simulink model "feng_unpack"  (R2012b)
settings: Solver=FixedStepDiscrete  SolverMode=SingleTasking  StartTime=0.0  StopTime=1500000  RelTol=1e-3
undefined symbols (not defined in the file or in its folder): Down, Up
libraries: xbsIndex_r4 x1511, simulink x1, xps_library x1
(part 3 of 13)

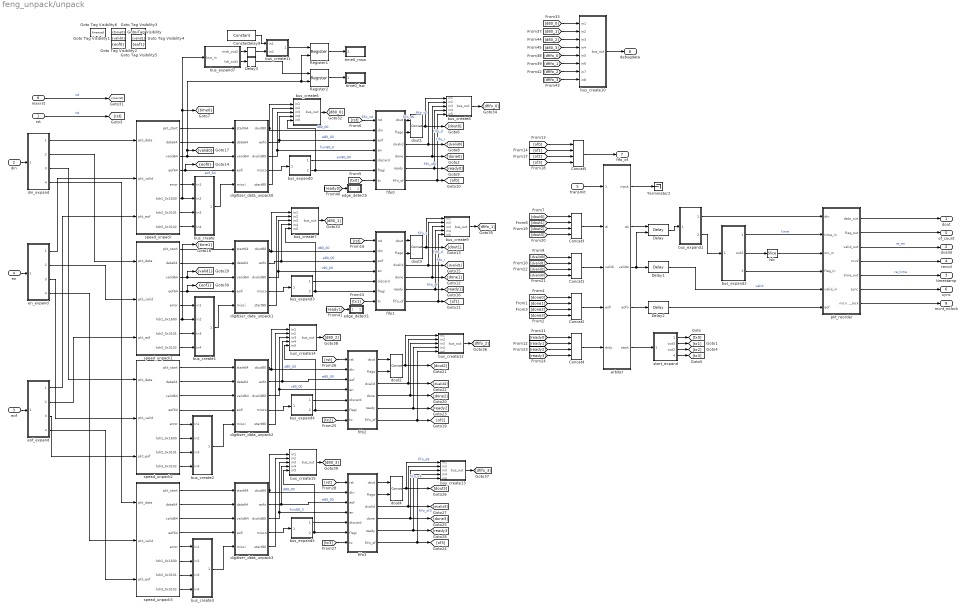
== system feng_unpack/unpack ==
  rst : Inport
  din : Inport  Port=2
  eof : Inport  Port=3
  en : Inport  Port=4
  transmit : Inport  Port=5
  maxrst : Inport  Port=6
  Concat{1..5} (5 alike) : xbsIndex_r4/Concat  num_inputs=4  dbl_ovrd=off  block_type=concat
  Constant : xbsIndex_r4/Constant  const=762.331  gui_display_data_type=Fixed-point  arith_type=Signed (2's comp)  n_bits=16  bin_pt=5  preci_type=Single  exp_width=8  frac_width=24  explicit_period=on  period=1  equ=P=C  opselect=C  inp2=PCIN>>17  opr=+  inp1=P  carry=CIN  dbl_ovrd=off  block_type=constant
  Delay : xbsIndex_r4/Delay  rst=off  infoeditControl=Selection of Reset will increase slice count due to use of real FFs and instead of SRLs  en=on  latency=1  dbl_ovrd=off  reg_retiming=on  block_type=delay
  Delay1 : xbsIndex_r4/Delay  rst=off  infoeditControl=Selection of Reset will increase slice count due to use of real FFs and instead of SRLs  en=off  latency=1  dbl_ovrd=off  reg_retiming=on  block_type=delay
  Delay2 : xbsIndex_r4/Delay  rst=off  infoeditControl=Selection of Reset will increase slice count due to use of real FFs and instead of SRLs  en=off  latency=1  dbl_ovrd=off  reg_retiming=on  block_type=delay
  Delay3 : xbsIndex_r4/Delay  rst=off  infoeditControl=Selection of Reset will increase slice count due to use of real FFs and instead of SRLs  en=off  latency=1  dbl_ovrd=off  reg_retiming=off  block_type=delay
  Delay9 : xbsIndex_r4/Delay  rst=off  infoeditControl=Selection of Reset will increase slice count due to use of real FFs and instead of SRLs  en=off  latency=1  dbl_ovrd=off  reg_retiming=off  block_type=delay
  Goto Tag Visibility : GotoTagVisibility  GotoTag=time0
  Goto Tag Visibility1 : GotoTagVisibility  GotoTag=valid0
  Goto Tag Visibility2 : GotoTagVisibility  GotoTag=eof0
  Goto Tag Visibility3 : GotoTagVisibility  GotoTag=time1
  Goto Tag Visibility4 : GotoTagVisibility  GotoTag=valid1
  Goto Tag Visibility5 : GotoTagVisibility  GotoTag=eof1
  Goto Tag Visibility6 : GotoTagVisibility  GotoTag=maxrst
  Register1 : xbsIndex_r4/Register  init=0  rst=off  en=on  dbl_ovrd=off  block_type=register
  Register2 : xbsIndex_r4/Register  init=0  rst=off  en=on  dbl_ovrd=off  block_type=register
  Terminator2 : Terminator
  arbiter : Subsystem  mask{n_inputs=4, n_bits_input=160 + n_bits_timestamp + n_bits_source + n_bits_of_count, mux_latency=1, preempt=1, n_bits_block_size=n_bits_packet_size-1, n_cycles_preempt=6}
      mask prompts: n_inputs "number of inputs"; n_bits_input "input bit widths"; mux_latency "mux latency"; preempt "preempt start of next block"; n_bits_block_size "data block size (2^?)"; n_cycles_preempt "clock cycles to preempt at"
      mask init:
      | set_param([gcb, '/eofi_mux'], ...
      |     'n_bits', 'ones(1, n_inputs)', ...
      |     'mux_latency', 'mux_latency', ...
      |     'cmplx', 'off', 'misc', 'off');
      | set_param([gcb, '/di_mux'], ...
      |     'n_bits', 'repmat(n_bits_input, 1, n_inputs)', ...
      |     'mux_latency', 'mux_latency', ...
      |     'cmplx', 'off', 'misc', 'off');
      | set_param([gcb, '/validi_mux'], ...
      |     'n_bits', 'ones(1, n_inputs)', ...
      |     'mux_latency', 'mux_latency', ...
      |     'cmplx', 'off', 'misc', 'off');
      | set_param([gcb, '/busy_edge_rep'], ...
      |     'replication', 'n_inputs', ...
      |     'misc', 'off');
  bus_create : Subsystem  AncestorBlock=casper_library_flow_control/bus_create  mask(bus_create){inputNum=4}
      mask prompts: inputNum "Number of inputs:"
      mask init:
      | bus_create_init(gcb,...
      |     'inputNum', inputNum);
  bus_create1 : Subsystem  AncestorBlock=casper_library_flow_control/bus_create  mask(bus_create){inputNum=4}
      mask prompts: inputNum "Number of inputs:"
      mask init:
      | bus_create_init(gcb,...
      |     'inputNum', inputNum);
  bus_create10 : Subsystem  AncestorBlock=casper_library_flow_control/bus_create  mask(bus_create){inputNum=8}
      mask prompts: inputNum "Number of inputs:"
      mask init:
      | bus_create_init(gcb,...
      |     'inputNum', inputNum);
  bus_create11 : Subsystem  AncestorBlock=casper_library_flow_control/bus_create  mask(bus_create){inputNum=2}
      mask prompts: inputNum "Number of inputs:"
      mask init:
      | bus_create_init(gcb,...
      |     'inputNum', inputNum);
  bus_create12 : Subsystem  AncestorBlock=casper_library_flow_control/bus_create  mask(bus_create){inputNum=5}
      mask prompts: inputNum "Number of inputs:"
      mask init:
      | bus_create_init(gcb,...
      |     'inputNum', inputNum);
  bus_create13 : Subsystem  AncestorBlock=casper_library_flow_control/bus_create  mask(bus_create){inputNum=5}
      mask prompts: inputNum "Number of inputs:"
      mask init:
      | bus_create_init(gcb,...
      |     'inputNum', inputNum);
  bus_create14 : Subsystem  AncestorBlock=casper_library_flow_control/bus_create  mask(bus_create){inputNum=5}
      mask prompts: inputNum "Number of inputs:"
      mask init:
      | bus_create_init(gcb,...
      |     'inputNum', inputNum);
  bus_create15 : Subsystem  AncestorBlock=casper_library_flow_control/bus_create  mask(bus_create){inputNum=5}
      mask prompts: inputNum "Number of inputs:"
      mask init:
      | bus_create_init(gcb,...
      |     'inputNum', inputNum);
  bus_create2 : Subsystem  AncestorBlock=casper_library_flow_control/bus_create  mask(bus_create){inputNum=4}
      mask prompts: inputNum "Number of inputs:"
      mask init:
      | bus_create_init(gcb,...
      |     'inputNum', inputNum);
  bus_create3 : Subsystem  AncestorBlock=casper_library_flow_control/bus_create  mask(bus_create){inputNum=4}
      mask prompts: inputNum "Number of inputs:"
      mask init:
      | bus_create_init(gcb,...
      |     'inputNum', inputNum);
  bus_create6 : Subsystem  AncestorBlock=casper_library_flow_control/bus_create  mask(bus_create){inputNum=5}
      mask prompts: inputNum "Number of inputs:"
      mask init:
      | bus_create_init(gcb,...
      |     'inputNum', inputNum);
  bus_create7 : Subsystem  AncestorBlock=casper_library_flow_control/bus_create  mask(bus_create){inputNum=5}
      mask prompts: inputNum "Number of inputs:"
      mask init:
      | bus_create_init(gcb,...
      |     'inputNum', inputNum);
  bus_create8 : Subsystem  AncestorBlock=casper_library_flow_control/bus_create  mask(bus_create){inputNum=5}
      mask prompts: inputNum "Number of inputs:"
      mask init:
      | bus_create_init(gcb,...
      |     'inputNum', inputNum);
  bus_create9 : Subsystem  AncestorBlock=casper_library_flow_control/bus_create  mask(bus_create){inputNum=5}
      mask prompts: inputNum "Number of inputs:"
      mask init:
      | bus_create_init(gcb,...
      |     'inputNum', inputNum);
  bus_expand0 : Subsystem  AncestorBlock=casper_library_flow_control/bus_expand  mask(bus_expand){mode=divisions of arbitrary size, outputNum=1, outputWidth=[1, sum([n_bits_timestamp, n_bits_source, n_bits_of_count])], outputBinaryPt=[0 0], outputArithmeticType=[2 0], show_format=on, outputToWorkspace=off, variablePrefix=out, outputToModelAsWell=on}
      mask prompts: outputNum "Number of outputs:"; outputWidth "Output width [msb ... lsb]:"; outputBinaryPt "Output binary point position [msb ... lsb]:"; outputArithmeticType "Output arithmetic type (ufix=0, fix=1, bool=2) [msb ... lsb]:"; show_format "Print format string?"; outputToWorkspace "Output to workspace?"; variablePrefix "Variable name prefix:"; outputToModelAsWell "Output to model as well?"
      mask help:
      | Expands a 'bus' made using a bus_create or Xilinx
      | concat block.
      | The input will be divided into the specified number
      | of outputs with the specified arithmetic types.
      | Divisions are made from most significant bit.
      mask init: same as feng_unpack/bus_expand10
      settings: AttributesFormatString=2 outputs: b,uf144.0,
      mask TypeOptions mode: divisions of equal size | divisions of arbitrary size
      mask Callback mode: bus_expand_callback();
      mask Callback outputWidth: bus_expand_callback();
      mask Callback outputToWorkspace: bus_expand_callback();
  bus_expand1 : Subsystem  AncestorBlock=casper_library_flow_control/bus_expand  mask(bus_expand){mode=divisions of arbitrary size, outputNum=1, outputWidth=[160, sum([n_bits_timestamp, n_bits_source, n_bits_of_count])], outputBinaryPt=[0 0], outputArithmeticType=[0 0], show_format=off, outputToWorkspace=off, variablePrefix=out, outputToModelAsWell=on}
      mask prompts: outputNum "Number of outputs:"; outputWidth "Output width [msb ... lsb]:"; outputBinaryPt "Output binary point position [msb ... lsb]:"; outputArithmeticType "Output arithmetic type (ufix=0, fix=1, bool=2) [msb ... lsb]:"; show_format "Print format string?"; outputToWorkspace "Output to workspace?"; variablePrefix "Variable name prefix:"; outputToModelAsWell "Output to model as well?"
      mask help:
      | Expands a 'bus' made using a bus_create or Xilinx
      | concat block.
      | The input will be divided into the specified number
      | of outputs with the specified arithmetic types.
      | Divisions are made from most significant bit.
      mask init: same as feng_unpack/bus_expand10
      settings: AttributesFormatString=2 outputs
      mask TypeOptions mode: divisions of equal size | divisions of arbitrary size
      mask Callback mode: bus_expand_callback();
      mask Callback outputWidth: bus_expand_callback();
      mask Callback outputToWorkspace: bus_expand_callback();
  bus_expand2 : Subsystem  AncestorBlock=casper_library_flow_control/bus_expand  mask(bus_expand){mode=divisions of arbitrary size, outputNum=1, outputWidth=[n_bits_timestamp, n_bits_source, n_bits_of_count], outputBinaryPt=[0 0 0], outputArithmeticType=[0 0 0], show_format=off, outputToWorkspace=off, variablePrefix=out, outputToModelAsWell=on}
      mask prompts: outputNum "Number of outputs:"; outputWidth "Output width [msb ... lsb]:"; outputBinaryPt "Output binary point position [msb ... lsb]:"; outputArithmeticType "Output arithmetic type (ufix=0, fix=1, bool=2) [msb ... lsb]:"; show_format "Print format string?"; outputToWorkspace "Output to workspace?"; variablePrefix "Variable name prefix:"; outputToModelAsWell "Output to model as well?"
      mask help:
      | Expands a 'bus' made using a bus_create or Xilinx
      | concat block.
      | The input will be divided into the specified number
      | of outputs with the specified arithmetic types.
      | Divisions are made from most significant bit.
      mask init: same as feng_unpack/bus_expand10
      settings: AttributesFormatString=3 outputs
      mask TypeOptions mode: divisions of equal size | divisions of arbitrary size
      mask Callback mode: bus_expand_callback();
      mask Callback outputWidth: bus_expand_callback();
      mask Callback outputToWorkspace: bus_expand_callback();
  bus_expand3 : Subsystem  AncestorBlock=casper_library_flow_control/bus_expand  mask(bus_expand){mode=divisions of arbitrary size, outputNum=1, outputWidth=[1, sum([n_bits_timestamp, n_bits_source, n_bits_of_count])], outputBinaryPt=[0 0], outputArithmeticType=[2 0], show_format=off, outputToWorkspace=off, variablePrefix=out, outputToModelAsWell=on}
      mask prompts: outputNum "Number of outputs:"; outputWidth "Output width [msb ... lsb]:"; outputBinaryPt "Output binary point position [msb ... lsb]:"; outputArithmeticType "Output arithmetic type (ufix=0, fix=1, bool=2) [msb ... lsb]:"; show_format "Print format string?"; outputToWorkspace "Output to workspace?"; variablePrefix "Variable name prefix:"; outputToModelAsWell "Output to model as well?"
      mask help:
      | Expands a 'bus' made using a bus_create or Xilinx
      | concat block.
      | The input will be divided into the specified number
      | of outputs with the specified arithmetic types.
      | Divisions are made from most significant bit.
      mask init: same as feng_unpack/bus_expand10
      settings: AttributesFormatString=2 outputs
      mask TypeOptions mode: divisions of equal size | divisions of arbitrary size
      mask Callback mode: bus_expand_callback();
      mask Callback outputWidth: bus_expand_callback();
      mask Callback outputToWorkspace: bus_expand_callback();
  bus_expand4 : Subsystem  AncestorBlock=casper_library_flow_control/bus_expand  mask(bus_expand){mode=divisions of arbitrary size, outputNum=1, outputWidth=[1, sum([n_bits_timestamp, n_bits_source, n_bits_of_count])], outputBinaryPt=[0 0], outputArithmeticType=[2 0], show_format=off, outputToWorkspace=off, variablePrefix=out, outputToModelAsWell=on}
      mask prompts: outputNum "Number of outputs:"; outputWidth "Output width [msb ... lsb]:"; outputBinaryPt "Output binary point position [msb ... lsb]:"; outputArithmeticType "Output arithmetic type (ufix=0, fix=1, bool=2) [msb ... lsb]:"; show_format "Print format string?"; outputToWorkspace "Output to workspace?"; variablePrefix "Variable name prefix:"; outputToModelAsWell "Output to model as well?"
      mask help:
      | Expands a 'bus' made using a bus_create or Xilinx
      | concat block.
      | The input will be divided into the specified number
      | of outputs with the specified arithmetic types.
      | Divisions are made from most significant bit.
      mask init: same as feng_unpack/bus_expand10
      settings: AttributesFormatString=2 outputs
      mask TypeOptions mode: divisions of equal size | divisions of arbitrary size
      mask Callback mode: bus_expand_callback();
      mask Callback outputWidth: bus_expand_callback();
      mask Callback outputToWorkspace: bus_expand_callback();
  bus_expand5 : Subsystem  AncestorBlock=casper_library_flow_control/bus_expand  mask(bus_expand){mode=divisions of arbitrary size, outputNum=1, outputWidth=[1, sum([n_bits_timestamp, n_bits_source, n_bits_of_count])], outputBinaryPt=[0 0], outputArithmeticType=[2 0], show_format=off, outputToWorkspace=off, variablePrefix=out, outputToModelAsWell=on}
      mask prompts: outputNum "Number of outputs:"; outputWidth "Output width [msb ... lsb]:"; outputBinaryPt "Output binary point position [msb ... lsb]:"; outputArithmeticType "Output arithmetic type (ufix=0, fix=1, bool=2) [msb ... lsb]:"; show_format "Print format string?"; outputToWorkspace "Output to workspace?"; variablePrefix "Variable name prefix:"; outputToModelAsWell "Output to model as well?"
      mask help:
      | Expands a 'bus' made using a bus_create or Xilinx
      | concat block.
      | The input will be divided into the specified number
      | of outputs with the specified arithmetic types.
      | Divisions are made from most significant bit.
      mask init: same as feng_unpack/bus_expand10
      settings: AttributesFormatString=2 outputs
      mask TypeOptions mode: divisions of equal size | divisions of arbitrary size
      mask Callback mode: bus_expand_callback();
      mask Callback outputWidth: bus_expand_callback();
      mask Callback outputToWorkspace: bus_expand_callback();
  bus_expand7 : Subsystem  AncestorBlock=casper_library_flow_control/bus_expand  mask(bus_expand){mode=divisions of arbitrary size, outputNum=1, outputWidth=[16 32], outputBinaryPt=[0 0], outputArithmeticType=[0 0], show_format=on, outputToWorkspace=off, variablePrefix=out, outputToModelAsWell=on}
      mask prompts: outputNum "Number of outputs:"; outputWidth "Output width [msb ... lsb]:"; outputBinaryPt "Output binary point position [msb ... lsb]:"; outputArithmeticType "Output arithmetic type (ufix=0, fix=1, bool=2) [msb ... lsb]:"; show_format "Print format string?"; outputToWorkspace "Output to workspace?"; variablePrefix "Variable name prefix:"; outputToModelAsWell "Output to model as well?"
      mask help:
      | Expands a 'bus' made using a bus_create or Xilinx
      | concat block.
      | The input will be divided into the specified number
      | of outputs with the specified arithmetic types.
      | Divisions are made from most significant bit.
      mask init: same as feng_unpack/bus_expand10
      settings: AttributesFormatString=2 outputs: uf16.0,uf32.0,
      mask TypeOptions mode: divisions of equal size | divisions of arbitrary size
      mask Callback mode: bus_expand_callback();
      mask Callback outputWidth: bus_expand_callback();
      mask Callback outputToWorkspace: bus_expand_callback();
  digitiser_data_unpack0 : Subsystem
  digitiser_data_unpack1 : Subsystem
  digitiser_data_unpack2 : Subsystem
  digitiser_data_unpack3 : Subsystem
  din_expand : Subsystem  AncestorBlock=casper_library_flow_control/bus_expand  mask(bus_expand){mode=divisions of equal size, outputNum=4, outputWidth=64, outputBinaryPt=0, outputArithmeticType=0, show_format=off, outputToWorkspace=off, variablePrefix=out, outputToModelAsWell=on}
      mask prompts: outputNum "Number of outputs:"; outputWidth "Output width:"; outputBinaryPt "Output binary point position:"; outputArithmeticType "Output arithmetic type (ufix=0, fix=1, bool=2):"; show_format "Print format string?"; outputToWorkspace "Output to workspace?"; variablePrefix "Variable name prefix:"; outputToModelAsWell "Output to model as well?"
      mask help:
      | Expands a 'bus' made using a bus_create or Xilinx
      | concat block.
      | The input will be divided into the specified number
      | of outputs with the specified arithmetic types.
      | Divisions are made from most significant bit.
      mask init: same as feng_unpack/bus_expand10
      settings: AttributesFormatString=4 outputs
      mask TypeOptions mode: divisions of equal size | divisions of arbitrary size
      mask Callback mode: bus_expand_callback();
      mask Callback outputWidth: bus_expand_callback();
      mask Callback outputToWorkspace: bus_expand_callback();
  dout{1..4} (4 alike) : xbsIndex_r4/Concat  num_inputs=2  dbl_ovrd=off  block_type=concat
  edge_detect1 : Subsystem  AncestorBlock=casper_library_misc/edge_detect  mask(edge_detect){edge=Rising, polarity=Active High, x_in=[0 0.08 0.08 0.16 0.16 0.24 0.24 0.32 0.32 0.4], y_in=[-1 -1  1  1  1  1  1  1  1  1], x_out=[0.6 0.68 0.68 0.76 0.76 0.84 0.84 0.92 0.92 1], y_out=[-1 -1  1  1 -1 -1 -1 -1 -1 -1]}
      mask prompts: edge "Edge Type"; polarity "Output Polarity"; x_in "Input X Positions"; y_in "Input Y Positions"; x_out "Output X Positions"; y_out "Output Y Positions"
      mask help: Output is active for one-cycle after each edge of the specified type (i.e. rising, falling or both).
      mask init: same as feng_unpack/edge_detect1
      settings: AttributesFormatString=|
      | rising edges
      | active high
      mask Help: Output is active for one-cycle after each edge of the specified type (i.e. rising, falling, or both).  Latency is zero.
      mask TypeOptions edge: Rising | Falling | Both
      mask TypeOptions polarity: Active High | Active Low
      mask Display:
      | plot(x_in_num,0.5+y_in_num*0.2);
      | plot(x_out_num,0.5+y_out_num*0.2);
  edge_detect5 : Subsystem  AncestorBlock=casper_library_misc/edge_detect  mask(edge_detect){edge=Rising, polarity=Active High, x_in=[0 0.08 0.08 0.16 0.16 0.24 0.24 0.32 0.32 0.4], y_in=[-1 -1  1  1  1  1  1  1  1  1], x_out=[0.6 0.68 0.68 0.76 0.76 0.84 0.84 0.92 0.92 1], y_out=[-1 -1  1  1 -1 -1 -1 -1 -1 -1]}
      mask prompts: edge "Edge Type"; polarity "Output Polarity"; x_in "Input X Positions"; y_in "Input Y Positions"; x_out "Output X Positions"; y_out "Output Y Positions"
      mask help: Output is active for one-cycle after each edge of the specified type (i.e. rising, falling or both).
      mask init: same as feng_unpack/edge_detect1
      settings: AttributesFormatString=|
      | rising edges
      | active high
      mask Help: Output is active for one-cycle after each edge of the specified type (i.e. rising, falling, or both).  Latency is zero.
      mask TypeOptions edge: Rising | Falling | Both
      mask TypeOptions polarity: Active High | Active Low
      mask Display:
      | plot(x_in_num,0.5+y_in_num*0.2);
      | plot(x_out_num,0.5+y_out_num*0.2);
  en_expand : Subsystem  AncestorBlock=casper_library_flow_control/bus_expand  mask(bus_expand){mode=divisions of equal size, outputNum=4, outputWidth=1, outputBinaryPt=0, outputArithmeticType=2, show_format=off, outputToWorkspace=off, variablePrefix=out, outputToModelAsWell=on}
      mask prompts: outputNum "Number of outputs:"; outputWidth "Output width:"; outputBinaryPt "Output binary point position:"; outputArithmeticType "Output arithmetic type (ufix=0, fix=1, bool=2):"; show_format "Print format string?"; outputToWorkspace "Output to workspace?"; variablePrefix "Variable name prefix:"; outputToModelAsWell "Output to model as well?"
      mask help:
      | Expands a 'bus' made using a bus_create or Xilinx
      | concat block.
      | The input will be divided into the specified number
      | of outputs with the specified arithmetic types.
      | Divisions are made from most significant bit.
      mask init: same as feng_unpack/bus_expand10
      settings: AttributesFormatString=4 outputs
      mask TypeOptions mode: divisions of equal size | divisions of arbitrary size
      mask Callback mode: bus_expand_callback();
      mask Callback outputWidth: bus_expand_callback();
      mask Callback outputToWorkspace: bus_expand_callback();
  eof_expand : Subsystem  AncestorBlock=casper_library_flow_control/bus_expand  mask(bus_expand){mode=divisions of equal size, outputNum=4, outputWidth=1, outputBinaryPt=0, outputArithmeticType=2, show_format=off, outputToWorkspace=off, variablePrefix=out, outputToModelAsWell=on}
      mask prompts: outputNum "Number of outputs:"; outputWidth "Output width:"; outputBinaryPt "Output binary point position:"; outputArithmeticType "Output arithmetic type (ufix=0, fix=1, bool=2):"; show_format "Print format string?"; outputToWorkspace "Output to workspace?"; variablePrefix "Variable name prefix:"; outputToModelAsWell "Output to model as well?"
      mask help:
      | Expands a 'bus' made using a bus_create or Xilinx
      | concat block.
      | The input will be divided into the specified number
      | of outputs with the specified arithmetic types.
      | Divisions are made from most significant bit.
      mask init: same as feng_unpack/bus_expand10
      settings: AttributesFormatString=4 outputs
      mask TypeOptions mode: divisions of equal size | divisions of arbitrary size
      mask Callback mode: bus_expand_callback();
      mask Callback outputWidth: bus_expand_callback();
      mask Callback outputToWorkspace: bus_expand_callback();
  fifo0 : Subsystem  mask{n_bits_din=80, n_bits_flag=sum([n_bits_timestamp, n_bits_source, n_bits_of_count]), scale_factor_bits=1, input_word_count_bits=n_bits_packet_size, bram_latency=bram_latency}
      mask prompts: n_bits_din "input data bit width"; n_bits_flag "flag bit width"; scale_factor_bits "output width scale factor (2^?)"; input_word_count_bits "max input word count (2^?)"; bram_latency "BRAM latency"
  fifo1 : Subsystem  mask{n_bits_din=80, n_bits_flag=sum([n_bits_timestamp, n_bits_source, n_bits_of_count]), scale_factor_bits=1, input_word_count_bits=n_bits_packet_size, bram_latency=bram_latency}
      mask prompts: n_bits_din "input data bit width"; n_bits_flag "flag bit width"; scale_factor_bits "output width scale factor (2^?)"; input_word_count_bits "max input word count (2^?)"; bram_latency "BRAM latency"
  fifo2 : Subsystem  mask{n_bits_din=80, n_bits_flag=sum([n_bits_timestamp, n_bits_source, n_bits_of_count]), scale_factor_bits=1, input_word_count_bits=n_bits_packet_size, bram_latency=bram_latency}
      mask prompts: n_bits_din "input data bit width"; n_bits_flag "flag bit width"; scale_factor_bits "output width scale factor (2^?)"; input_word_count_bits "max input word count (2^?)"; bram_latency "BRAM latency"
  fifo3 : Subsystem  mask{n_bits_din=80, n_bits_flag=sum([n_bits_timestamp, n_bits_source, n_bits_of_count]), scale_factor_bits=1, input_word_count_bits=n_bits_packet_size, bram_latency=bram_latency}
      mask prompts: n_bits_din "input data bit width"; n_bits_flag "flag bit width"; scale_factor_bits "output width scale factor (2^?)"; input_word_count_bits "max input word count (2^?)"; bram_latency "BRAM latency"
  lsb : xbsIndex_r4/Slice  nbits=1  boolean_output=off  mode=Lower Bit Location + Width  bit1=0  base1=MSB of Input  bit0=0  base0=LSB of Input  dbl_ovrd=off  block_type=slice
  pkt_reorder : Subsystem  mask{window_bits=n_bits_buffer, window_size_bits=n_bits_packet_size - 1, n_bits_din=80, n_bits_flag=n_bits_of_count, n_bits_timestamp=n_bits_timestamp}
      mask prompts: window_bits "Number of Windows to Buffer (2^?)"; window_size_bits "Window size (2^?)"; n_bits_din "Data bit width in"; n_bits_flag "Flag bit width in"; n_bits_timestamp "Timestamp bit width"
      mask init:
      | fmtstr = sprintf('Buffer space: 2^%i words', window_bits+window_size_bits);
      | set_param(gcb, 'AttributesFormatString', fmtstr);
      settings: AttributesFormatString=Buffer space: 2^11 words
  spead_unpack : Subsystem  Tag=casper:spead_unpack  AncestorBlock=casper_library_communications/spead_unpack  mask(spead_unpack_mask){payload_length=640, header_ids=[5632 12545 12546], spead_msw=64, spead_lsw=48, spead_version=4, combine_errors=on}
      mask prompts: payload_length "Payload length in 64-bit words"; header_ids "SPEAD header IDs (decimal)"; spead_msw "SPEAD Flavour (MSw)"; spead_lsw "SPEAD Flavour (LSw)"; spead_version "SPEAD version"; combine_errors "Combine error flags"
      mask help: This block receives a 64-bit-word stream that contains a SPEAD stream. It checks the SPEAD headers are being correctly received. It presents the user with all headers on the first valid cycle of data along with a flag to indicate a header or packet-length error.
      mask init:
      | spead_unpack_init(gcb)
  spead_unpack1 : Subsystem  Tag=casper:spead_unpack  AncestorBlock=casper_library_communications/spead_unpack  mask(spead_unpack_mask){payload_length=640, header_ids=[5632 12545 12546], spead_msw=64, spead_lsw=48, spead_version=4, combine_errors=on}
      mask prompts: payload_length "Payload length in 64-bit words"; header_ids "SPEAD header IDs (decimal)"; spead_msw "SPEAD Flavour (MSw)"; spead_lsw "SPEAD Flavour (LSw)"; spead_version "SPEAD version"; combine_errors "Combine error flags"
      mask help: This block receives a 64-bit-word stream that contains a SPEAD stream. It checks the SPEAD headers are being correctly received. It presents the user with all headers on the first valid cycle of data along with a flag to indicate a header or packet-length error.
      mask init:
      | spead_unpack_init(gcb)
  spead_unpack2 : Subsystem  Tag=casper:spead_unpack  AncestorBlock=casper_library_communications/spead_unpack  mask(spead_unpack_mask){payload_length=640, header_ids=[5632 12545 12546], spead_msw=64, spead_lsw=48, spead_version=4, combine_errors=on}
      mask prompts: payload_length "Payload length in 64-bit words"; header_ids "SPEAD header IDs (decimal)"; spead_msw "SPEAD Flavour (MSw)"; spead_lsw "SPEAD Flavour (LSw)"; spead_version "SPEAD version"; combine_errors "Combine error flags"
      mask help: This block receives a 64-bit-word stream that contains a SPEAD stream. It checks the SPEAD headers are being correctly received. It presents the user with all headers on the first valid cycle of data along with a flag to indicate a header or packet-length error.
      mask init:
      | spead_unpack_init(gcb)
  spead_unpack3 : Subsystem  Tag=casper:spead_unpack  AncestorBlock=casper_library_communications/spead_unpack  mask(spead_unpack_mask){payload_length=640, header_ids=[5632 12545 12546], spead_msw=64, spead_lsw=48, spead_version=4, combine_errors=on}
      mask prompts: payload_length "Payload length in 64-bit words"; header_ids "SPEAD header IDs (decimal)"; spead_msw "SPEAD Flavour (MSw)"; spead_lsw "SPEAD Flavour (LSw)"; spead_version "SPEAD version"; combine_errors "Combine error flags"
      mask help: This block receives a 64-bit-word stream that contains a SPEAD stream. It checks the SPEAD headers are being correctly received. It presents the user with all headers on the first valid cycle of data along with a flag to indicate a header or packet-length error.
      mask init:
      | spead_unpack_init(gcb)
  start_expand : Subsystem  AncestorBlock=casper_library_flow_control/bus_expand  mask(bus_expand){mode=divisions of equal size, outputNum=4, outputWidth=1, outputBinaryPt=0, outputArithmeticType=2, show_format=off, outputToWorkspace=off, variablePrefix=out, outputToModelAsWell=on}
      mask prompts: outputNum "Number of outputs:"; outputWidth "Output width:"; outputBinaryPt "Output binary point position:"; outputArithmeticType "Output arithmetic type (ufix=0, fix=1, bool=2):"; show_format "Print format string?"; outputToWorkspace "Output to workspace?"; variablePrefix "Variable name prefix:"; outputToModelAsWell "Output to model as well?"
      mask help:
      | Expands a 'bus' made using a bus_create or Xilinx
      | concat block.
      | The input will be divided into the specified number
      | of outputs with the specified arithmetic types.
      | Divisions are made from most significant bit.
      mask init: same as feng_unpack/bus_expand10
      settings: AttributesFormatString=4 outputs
      mask TypeOptions mode: divisions of equal size | divisions of arbitrary size
      mask Callback mode: bus_expand_callback();
      mask Callback outputWidth: bus_expand_callback();
      mask Callback outputToWorkspace: bus_expand_callback();
  time0_lsw : Subsystem  Tag=xps:sw_reg  AncestorBlock=xps_library/software register  mask(swreg){mode=one value, io_dir=To Processor, io_delay=0, sample_period=1, names=reg, bitwidths=32, arith_types=0, bin_pts=0, sim_port=off, show_format=off}
      mask prompts: io_dir "I/O direction"; io_delay "I/O delay"; sample_period "Sample period"; names "Name:"; bitwidths "Bitwidth:"; arith_types "Type (ufix=0, fix=1, bool=2):"; bin_pts "Binary pt:"; sim_port "Provide sim input/output?"; show_format "Print format string?"
      mask init:
      | swreg_init(gcb)
      settings: AttributesFormatString=1output
      mask TypeOptions mode: one value | fields of equal size | fields of arbitrary size
      mask Callback mode: swreg_cb(gcb);
      mask TypeOptions io_dir: To Processor | From Processor
      mask Callback io_dir:
      | mask_enables = get_param(gcb, 'MaskEnables');
      | mask_names = get_param(gcb, 'MaskNames');
      | if strcmp(get_param(gcb, 'io_dir'), 'To Processor'),
      |     mask_enables{ismember(mask_names, 'sample_period')} = 'off';
      | else
      |     mask_enables{ismember(mask_names, 'sample_period')} = 'on';
      | end
      | set_param(gcb, 'MaskEnables', mask_enables);
      mask Callback bitwidths:
      | blk = gcb;
      | mode = get_param(blk, 'mode');
      | current_widths = eval(get_param(blk, 'bitwidths'));
      | if (strcmp(mode, 'one value') || strcmp(mode, 'fields of equal size')) && (length(current_widths) > 1),
      |     error('Only one width may be specified for this mode.');
      | elseif strcmp(mode, 'fields of arbitrary size')
      |     current_names = textscan(strtrim(strrep(strrep(get_param(blk, 'names'), ']', ''), '[', '')), '%s');
      |     current_names = current_names{1};
      |     numios = length(current_names);
      |     if length(current_widths) ~= numios,
      |         error('%d field names specified, but %d widths?', numios, length(current_widths));
      |     end
      | end
      | total_width = 0;
      | for ctr = 1 : length(current_widths),
      |     total_width = total_width + current_widths(ctr);
      | end
      | if total_width > 32,
      |     error('Total width must be 32 or less, set to %d.', total_width);
      | end
      mask Callback arith_types:
      | blk = gcb;
      | mode = get_param(blk, 'mode');
      | current_types = eval(get_param(blk, 'arith_types'));
      | numios = length(current_types);
      | if (strcmp(mode, 'one value') || strcmp(mode, 'fields of equal size')) && (length(current_types) > 1),
      |     error('Only one type may be specified for this mode.');
      | elseif strcmp(mode, 'fields of arbitrary size')
      |     current_names = textscan(strtrim(strrep(strrep(get_param(blk, 'names'), ']', ''), '[', '')), '%s');
      |     current_names = current_names{1};
      |     numios = length(current_names);
      |     if length(current_types) ~= numios,
      |         error('%d field names specified, but %d types?', numios, length(current_types));
      |     end
      | end
      | problem = 0;
      | for ctr = 1 : numios,
      |     t = current_types(ctr);
      |     if (t < 0) || (t > 2),
      |         problem = t;
      |         ctr = numios + 1;
      |     end
      | end
      | if problem ~= 0,
      |     error('Type cannot be %i, must be 0, 1 or 2.', problem);
      | end
      mask Callback bin_pts:
      | blk = gcb;
      | mode = get_param(blk, 'mode');
      | current_bins = eval(get_param(blk, 'bin_pts'));
      | if (strcmp(mode, 'one value') || strcmp(mode, 'fields of equal size')) && (length(current_bins) > 1),
      |     error('Only one binary pt may be specified for this mode.');
      | elseif strcmp(mode, 'fields of arbitrary size')
      |     current_names = textscan(strtrim(strrep(strrep(get_param(blk, 'names'), ']', ''), '[', '')), '%s');
      |     current_names = current_names{1};
      |     numios = length(current_names);
      |     if length(current_bins) ~= numios,
      |         error('%d field names specified, but %d binary pts?', numios, length(current_bins));
      |     end
      | end
  time0_msw : Subsystem  Tag=xps:sw_reg  AncestorBlock=xps_library/software register  mask(swreg){mode=one value, io_dir=To Processor, io_delay=0, sample_period=1, names=reg, bitwidths=32, arith_types=0, bin_pts=0, sim_port=off, show_format=off}
      mask prompts: io_dir "I/O direction"; io_delay "I/O delay"; sample_period "Sample period"; names "Name:"; bitwidths "Bitwidth:"; arith_types "Type (ufix=0, fix=1, bool=2):"; bin_pts "Binary pt:"; sim_port "Provide sim input/output?"; show_format "Print format string?"
      mask init:
      | swreg_init(gcb)
      settings: AttributesFormatString=1output
      mask TypeOptions mode: one value | fields of equal size | fields of arbitrary size
      mask Callback mode: swreg_cb(gcb);
      mask TypeOptions io_dir: To Processor | From Processor
      mask Callback io_dir:
      | mask_enables = get_param(gcb, 'MaskEnables');
      | mask_names = get_param(gcb, 'MaskNames');
      | if strcmp(get_param(gcb, 'io_dir'), 'To Processor'),
      |     mask_enables{ismember(mask_names, 'sample_period')} = 'off';
      | else
      |     mask_enables{ismember(mask_names, 'sample_period')} = 'on';
      | end
      | set_param(gcb, 'MaskEnables', mask_enables);
      mask Callback bitwidths:
      | blk = gcb;
      | mode = get_param(blk, 'mode');
      | current_widths = eval(get_param(blk, 'bitwidths'));
      | if (strcmp(mode, 'one value') || strcmp(mode, 'fields of equal size')) && (length(current_widths) > 1),
      |     error('Only one width may be specified for this mode.');
      | elseif strcmp(mode, 'fields of arbitrary size')
      |     current_names = textscan(strtrim(strrep(strrep(get_param(blk, 'names'), ']', ''), '[', '')), '%s');
      |     current_names = current_names{1};
      |     numios = length(current_names);
      |     if length(current_widths) ~= numios,
      |         error('%d field names specified, but %d widths?', numios, length(current_widths));
      |     end
      | end
      | total_width = 0;
      | for ctr = 1 : length(current_widths),
      |     total_width = total_width + current_widths(ctr);
      | end
      | if total_width > 32,
      |     error('Total width must be 32 or less, set to %d.', total_width);
      | end
      mask Callback arith_types:
      | blk = gcb;
      | mode = get_param(blk, 'mode');
      | current_types = eval(get_param(blk, 'arith_types'));
      | numios = length(current_types);
      | if (strcmp(mode, 'one value') || strcmp(mode, 'fields of equal size')) && (length(current_types) > 1),
      |     error('Only one type may be specified for this mode.');
      | elseif strcmp(mode, 'fields of arbitrary size')
      |     current_names = textscan(strtrim(strrep(strrep(get_param(blk, 'names'), ']', ''), '[', '')), '%s');
      |     current_names = current_names{1};
      |     numios = length(current_names);
      |     if length(current_types) ~= numios,
      |         error('%d field names specified, but %d types?', numios, length(current_types));
      |     end
      | end
      | problem = 0;
      | for ctr = 1 : numios,
      |     t = current_types(ctr);
      |     if (t < 0) || (t > 2),
      |         problem = t;
      |         ctr = numios + 1;
      |     end
      | end
      | if problem ~= 0,
      |     error('Type cannot be %i, must be 0, 1 or 2.', problem);
      | end
      mask Callback bin_pts:
      | blk = gcb;
      | mode = get_param(blk, 'mode');
      | current_bins = eval(get_param(blk, 'bin_pts'));
      | if (strcmp(mode, 'one value') || strcmp(mode, 'fields of equal size')) && (length(current_bins) > 1),
      |     error('Only one binary pt may be specified for this mode.');
      | elseif strcmp(mode, 'fields of arbitrary size')
      |     current_names = textscan(strtrim(strrep(strrep(get_param(blk, 'names'), ']', ''), '[', '')), '%s');
      |     current_names = current_names{1};
      |     numios = length(current_names);
      |     if length(current_bins) ~= numios,
      |         error('%d field names specified, but %d binary pts?', numios, length(current_bins));
      |     end
      | end
  dout : Outport
  dvalid : Outport  Port=2
  timestamp : Outport  Port=3
  recvd : Outport  Port=4
  of_count : Outport  Port=5
  sync : Outport  Port=6
  fifo_of : Outport  Port=7
  debugdata : Outport  Port=8
  mcnt_nolock : Outport  Port=9
  tag scope: eof0=scoped, eof1=scoped, maxrst=scoped, time0=scoped, time1=scoped, valid0=scoped, valid1=scoped
  wires:
  Delay2/1 -> pkt_reorder/6(eof)
  Delay1/1 -> pkt_reorder/5(valid_in)  "valid"
  Delay/1 -> bus_expand1/1(bus_in)
  arbiter/4(eofo) -> Delay2/1
  arbiter/3(valido) -> Delay/2, Delay1/1
  arbiter/2(do) -> Delay/1
  eof_expand/4(lsb_out1) -> spead_unpack3/3(pkt_eof)
  eof_expand/3(out2) -> spead_unpack2/3(pkt_eof)
  eof_expand/2(out3) -> spead_unpack1/3(pkt_eof)
  eof_expand/1(msb_out4) -> spead_unpack/3(pkt_eof)
  en_expand/4(lsb_out1) -> spead_unpack3/2(pkt_valid)
  en_expand/3(out2) -> spead_unpack2/2(pkt_valid)
  en_expand/2(out3) -> spead_unpack1/2(pkt_valid)
  en_expand/1(msb_out4) -> spead_unpack/2(pkt_valid)
  din_expand/4(lsb_out1) -> spead_unpack3/1(pkt_data)
  din_expand/3(out2) -> spead_unpack2/1(pkt_data)
  din_expand/2(out3) -> spead_unpack1/1(pkt_data)
  din_expand/1(msb_out4) -> spead_unpack/1(pkt_data)
  spead_unpack/8(hdr3_0x3102) -> bus_create/4(in4)
  spead_unpack/7(hdr2_0x3101) -> bus_create/3(in3)
  spead_unpack/5(error) -> bus_create/1(in1)
  lsb/1 -> pkt_reorder/3(src_in)
  bus_expand2/2(out2) -> lsb/1
  fifo3/6(fifo_of) -> bus_create13/5(in5), [of3]  "fifo_of3"
  fifo3/5(ready) -> bus_create13/4(in4), [ready3]
  fifo3/4(done) -> bus_create13/3(in3), [done3]
  fifo3/3(dvalid) -> bus_create13/2(in2), [dvalid3]  "fifo_v3"
  dout4/1 -> bus_create13/1(in1), [dout3]  "fifo_d3"
  fifo3/2(flago) -> dout4/2
  fifo3/1(dout) -> dout4/1
  bus_expand5/2(lsb_out1) -> bus_create15/5(in5), fifo3/6(flagi)
  bus_expand5/1(msb_out2) -> fifo3/5(discard)
  digitiser_data_unpack3/3(dvalid80) -> bus_create15/3(in3), fifo3/4(en)  "fvin80_3"
  digitiser_data_unpack3/2(eofo) -> fifo3/3(eof), bus_create15/4(in4)  "e80_00"
  digitiser_data_unpack3/4(misco) -> bus_expand5/1(bus_in)
  digitiser_data_unpack3/1(dout80) -> bus_create15/1(in1), fifo3/2(din)  "d80_00"
  [rst] -> fifo3/1(rst)
  [tx3] -> fifo3/7(tx)
  fifo2/6(fifo_of) -> bus_create12/5(in5), [of2]
  fifo2/5(ready) -> bus_create12/4(in4), [ready2]
  fifo2/4(done) -> bus_create12/3(in3), [done2]
  fifo2/3(dvalid) -> bus_create12/2(in2), [dvalid2]
  dout2/1 -> bus_create12/1(in1), [dout2]
  dout3/1 -> [dout1], bus_create9/1(in1)
  fifo1/2(flago) -> dout3/2
  fifo1/1(dout) -> dout3/1
  fifo0/2(flago) -> dout1/2
  fifo0/1(dout) -> dout1/1  "fifo_d0"
  fifo2/2(flago) -> dout2/2
  fifo2/1(dout) -> dout2/1
  bus_expand4/2(lsb_out1) -> bus_create14/5(in5), fifo2/6(flagi)
  bus_expand4/1(msb_out2) -> fifo2/5(discard)
  digitiser_data_unpack2/3(dvalid80) -> bus_create14/3(in3), fifo2/4(en)  "v80_00"
  digitiser_data_unpack2/2(eofo) -> bus_create14/4(in4), fifo2/3(eof)  "e80_00"
  digitiser_data_unpack2/4(misco) -> bus_expand4/1(bus_in)
  digitiser_data_unpack2/1(dout80) -> bus_create14/1(in1), fifo2/2(din)  "d80_00"
  [rst] -> fifo2/1(rst)
  [tx2] -> fifo2/7(tx)
  fifo1/6(fifo_of) -> bus_create9/5(in5), [of1]  "fifo_of"
  fifo1/5(ready) -> [ready1], bus_create9/4(in4)  "fifo_r"
  fifo1/4(done) -> [done1], bus_create9/3(in3)  "fifo_d"
  fifo1/3(dvalid) -> [dvalid1], bus_create9/2(in2)  "fifo_v"
  bus_expand3/2(lsb_out1) -> bus_create7/5(in5), fifo1/6(flagi)
  bus_expand3/1(msb_out2) -> fifo1/5(discard)
  digitiser_data_unpack1/3(dvalid80) -> bus_create7/3(in3), fifo1/4(en)  "v80_00"
  digitiser_data_unpack1/2(eofo) -> bus_create7/4(in4), fifo1/3(eof)  "e80_00"
  digitiser_data_unpack1/4(misco) -> bus_expand3/1(bus_in)
  digitiser_data_unpack1/1(dout80) -> bus_create7/1(in1), fifo1/2(din)  "d80_00"
  [rst] -> fifo1/1(rst)
  bus_create3/1(bus_out) -> digitiser_data_unpack3/5(misci)
  spead_unpack3/8(hdr3_0x3102) -> bus_create3/4(in4)
  spead_unpack3/7(hdr2_0x3101) -> bus_create3/3(in3)
  spead_unpack3/6(hdr1_0x1600) -> bus_create3/2(in2)
  spead_unpack3/5(error) -> bus_create3/1(in1)
  spead_unpack3/4(eof64) -> digitiser_data_unpack3/4(eofi)
  spead_unpack3/3(valid64) -> digitiser_data_unpack3/3(valid64)
  spead_unpack3/2(data64) -> digitiser_data_unpack3/2(data64)
  bus_create2/1(bus_out) -> digitiser_data_unpack2/5(misci)
  spead_unpack2/8(hdr3_0x3102) -> bus_create2/4(in4)
  spead_unpack2/7(hdr2_0x3101) -> bus_create2/3(in3)
  spead_unpack2/6(hdr1_0x1600) -> bus_create2/2(in2)
  spead_unpack2/5(error) -> bus_create2/1(in1)
  spead_unpack2/4(eof64) -> digitiser_data_unpack2/4(eofi)
  spead_unpack2/3(valid64) -> digitiser_data_unpack2/3(valid64)
  spead_unpack2/2(data64) -> digitiser_data_unpack2/2(data64)
  bus_create1/1(bus_out) -> digitiser_data_unpack1/5(misci)
  spead_unpack1/8(hdr3_0x3102) -> bus_create1/4(in4)
  spead_unpack1/7(hdr2_0x3101) -> bus_create1/3(in3)
  spead_unpack1/6(hdr1_0x1600) -> [time1], bus_create1/2(in2)
  spead_unpack1/5(error) -> bus_create1/1(in1)
  spead_unpack1/4(eof64) -> [eof1], digitiser_data_unpack1/4(eofi)
  spead_unpack1/3(valid64) -> [valid1], digitiser_data_unpack1/3(valid64)
  spead_unpack1/2(data64) -> digitiser_data_unpack1/2(data64)
  bus_expand0/2(lsb_out1) -> bus_create6/5(in5), fifo0/6(flagi)
  bus_expand0/1(msb_out2) -> fifo0/5(discard)  "err80_00"
  bus_create/1(bus_out) -> digitiser_data_unpack0/5(misci)
  spead_unpack/4(eof64) -> [eof0], digitiser_data_unpack0/4(eofi)  "eof_64"
  spead_unpack/2(data64) -> digitiser_data_unpack0/2(data64)
  spead_unpack3/1(pkt_start) -> digitiser_data_unpack3/1(start64)
  spead_unpack2/1(pkt_start) -> digitiser_data_unpack2/1(start64)
  spead_unpack1/1(pkt_start) -> digitiser_data_unpack1/1(start64)
  spead_unpack/1(pkt_start) -> digitiser_data_unpack0/1(start64)
  bus_expand2/3(lsb_out1) -> pkt_reorder/4(flag_in)
  bus_expand2/1(msb_out3) -> pkt_reorder/2(time_in)  "time"
  bus_expand1/2(lsb_out1) -> bus_expand2/1(bus_in)
  bus_expand1/1(msb_out2) -> pkt_reorder/1(din)
  digitiser_data_unpack0/3(dvalid80) -> bus_create6/3(in3), fifo0/4(en)  "fvin80_0"
  digitiser_data_unpack0/2(eofo) -> bus_create6/4(in4), fifo0/3(eof)  "e80_00"
  digitiser_data_unpack0/4(misco) -> bus_expand0/1(bus_in)
  digitiser_data_unpack0/1(dout80) -> bus_create6/1(in1), fifo0/2(din)  "d80_00"
  eof/1 -> eof_expand/1(bus_in)
  en/1 -> en_expand/1(bus_in)
  din/1 -> din_expand/1(bus_in)
  [rst] -> fifo0/1(rst)  "fifo_rst"
  rst/1 -> [rst]  "rst"
  [of3] -> Concat5/4
  [of2] -> Concat5/3
  [of1] -> Concat5/2
  [of0] -> Concat5/1
  arbiter/1(input) -> Terminator2/1
  [ready3] -> Concat4/4
  [ready2] -> Concat4/3
  [dvalid3] -> Concat1/4
  [dvalid2] -> Concat1/3
  [dout3] -> Concat3/4
  [dout2] -> Concat3/3
  Concat5/1 -> fifo_of/1
  [ready1] -> Concat4/2
  [ready0] -> Concat4/1
  [dvalid1] -> Concat1/2
  [dvalid0] -> Concat1/1
  [dout1] -> Concat3/2
  [dout0] -> Concat3/1
  [done2] -> Concat2/3
  [done1] -> Concat2/2
  [done3] -> Concat2/4
  [done0] -> Concat2/1
  start_expand/4(lsb_out1) -> [tx3]
  start_expand/3(out2) -> [tx2]
  start_expand/2(out3) -> [tx1]
  start_expand/1(msb_out4) -> [tx0]
  transmit/1 -> arbiter/1(transmit)
  Concat1/1 -> arbiter/3(validi)
  Concat3/1 -> arbiter/2(di)
  Concat2/1 -> arbiter/4(eofi)
  Concat4/1 -> arbiter/5(drdy)
  arbiter/5(start) -> start_expand/1(bus_in)
  fifo0/6(fifo_of) -> bus_create8/5(in5), [of0]  "fifo_of0"
  fifo0/5(ready) -> [ready0], bus_create8/4(in4)  "fifo_r"
  fifo0/3(dvalid) -> [dvalid0], bus_create8/2(in2)  "fifo_v0"
  dout1/1 -> [dout0], bus_create8/1(in1)
  fifo0/4(done) -> [done0], bus_create8/3(in3)  "fifo_d"
  maxrst/1 -> [maxrst]  "rst"
  bus_create6/1(bus_out) -> [d80_0]
  bus_create8/1(bus_out) -> [dfifo_0]
  bus_create9/1(bus_out) -> [dfifo_1]
  bus_create10/1(bus_out) -> debugdata/1
  spead_unpack/6(hdr1_0x1600) -> bus_expand7/1(bus_in), [time0], bus_create/2(in2)
  spead_unpack/3(valid64) -> Register1/2, Register2/2, [valid0], digitiser_data_unpack0/3(valid64)
  bus_expand7/1(msb_out2) -> Delay9/1
  bus_expand7/2(lsb_out1) -> Delay3/1
  Delay9/1 -> bus_create11/2(in2)
  Constant/1 -> bus_create11/1(in1)
  bus_create11/1(bus_out) -> Register1/1
  Register1/1 -> time0_msw/1(out_reg)
  Register2/1 -> time0_lsw/1(out_reg)
  Delay3/1 -> Register2/1
  digitiser_data_unpack0/5(start80) -> bus_create6/2(in2)
  bus_create7/1(bus_out) -> [d80_1]
  digitiser_data_unpack1/5(start80) -> bus_create7/2(in2)
  [ready0] -> edge_detect5/1(in)
  [ready1] -> edge_detect1/1(in)
  pkt_reorder/1(data_out) -> dout/1
  pkt_reorder/2(flag_out) -> of_count/1
  pkt_reorder/3(valid_out) -> dvalid/1  "re_en"
  pkt_reorder/4(rcvd) -> recvd/1
  pkt_reorder/5(time_out) -> timestamp/1  "re_time"
  pkt_reorder/6(sync) -> sync/1
  pkt_reorder/7(mcnt_no_lock) -> mcnt_nolock/1
  [tx0] -> fifo0/7(tx)
  [tx1] -> fifo1/7(tx)
  bus_create12/1(bus_out) -> [dfifo_2]
  bus_create13/1(bus_out) -> [dfifo_3]
  bus_create14/1(bus_out) -> [d80_2]
  bus_create15/1(bus_out) -> [d80_3]
  digitiser_data_unpack2/5(start80) -> bus_create14/2(in2)
  digitiser_data_unpack3/5(start80) -> bus_create15/2(in2)
  [d80_0] -> bus_create10/1(in1)
  [d80_1] -> bus_create10/2(in2)
  [d80_2] -> bus_create10/3(in3)
  [d80_3] -> bus_create10/4(in4)
  [dfifo_1] -> bus_create10/6(in6)
  [dfifo_2] -> bus_create10/7(in7)
  [dfifo_3] -> bus_create10/8(in8)
  [dfifo_0] -> bus_create10/5(in5)
